simulink model "SVC_Simulation_V2"  (R2024a)
settings: Solver=FixedStepAuto  StartTime=0.0  StopTime=0.6  FixedStep=Ts  MaxStep=1e-5  RelTol=1e-4  AbsTol=1e-4
PreLoadFcn:
  | Ts=50e-6;
model workspace (MAT data in the model file):
  Ki : Simulink.Parameter (value not decoded)
  Kp = 0
symbols that are objects in the model workspace (value not decoded): Ki
undefined symbols (not defined in the file or in its folder): D1, Delta, DiscIntNeverNeededParam, find_system
libraries: spsSampleandHoldLib x24, spsThyristorLib x24, spsEdgeDetectorLib x12, spsSeriesRLCBranchLib x12, spsParallelRLCBranchLib x9, spsBistableLib x3, spsMeanVariableFrequencyLib x3, spsSecondOrderFilterLib x3, spsMultimeterLib x3, spsCurrentMeasurementLib x2, spsThreePhaseVIMeasurementLib x2, spsThreePhaseSeriesRLCLoadLib x1
(part 2 of 3)

== system SVC_Simulation_V2/SVC Controller/Firing Unit/Firing Unit BC ==
  note: PLL
      | sync on
      | pos. peak
      | of input
  note: Generate firing
      | pulses for TSC3
  note: Generate firing
      | pulse for TCR +
  note: Generate firing
      | pulse for TCR -
  note: Generate firing
      | pulses for TSC2
  note: Generate firing
      | pulses for TSC1
  note: Generate square-wave lagging Input
      | voltage by 90 degrees and pulses (width of
      | one sample) for positive (Sync +)
      | and negative (Sync -) transition
  note: Compute number
      | of samples per cycle
  note: Input
      | voltage
  V : Inport  PortDimensions=1
  Alpha : Inport  Port=2  PortDimensions=1
  TSC1_On : Inport  Port=3  PortDimensions=1
  TSC2_On : Inport  Port=4  PortDimensions=1
  TSC3_On : Inport  Port=5  PortDimensions=1
  BL2 : Subsystem
  BL3 : Subsystem
  Correction for delay : Gain  Gain=Nstep*Ts*2*pi  SaturateOnIntegerOverflow=on  OutDataTypeStr=Inherit: Same as input  ParamDataTypeStr=Inherit: Same as input
  Logical Operator2 : Logic  Operator=NOT  Inputs=3
  "PLL sync on positive peak " : Subsystem  mask(Discrete 1-phase PLL){Par_Init=[PhaseInit FreqInit], ParK=[120 2800], Ts=Ts}
      mask prompts: Par_Init "Initial input:[ Phase(degrees)   Frequency(Hz) ]"; ParK "Regulator gains [ Kp  Ki ]"; Ts "Sample time:"
      mask help:
      | This Phase Locked Loop (PLL) system can be used  to synchronize on a variable frequency sinusoidal signal.
      |
      | Input 1: Normalized input signal V(pu)
      mask init:
      | Kp=ParK(1);
      | Ki=ParK(2);
      | Phase_Init=Par_Init(1);
      | Finit=Par_Init(2);
  Sum : Sum  InputSameDT=on  SaturateOnIntegerOverflow=on  OutDataTypeStr=Inherit: Same as first input
  TCR Pulse Generatorr : Subsystem  mask{Ts=Ts}
      mask prompts: Ts "Sample time:"
  TCR Pulse Generatorr1 : Subsystem  mask{Ts=Ts}
      mask prompts: Ts "Sample time:"
  TCS Pulse Generator : Subsystem
  TCS Pulse Generator1 : Subsystem
  TCS Pulse Generator2 : Subsystem
  Trigonometric Function6 : Trigonometry
  TCR + : Outport  VectorParamsAs1DForOutWhenUnconnected=off
  TCR - : Outport  Port=2  VectorParamsAs1DForOutWhenUnconnected=off
  TSC1 + : Outport  Port=3  VectorParamsAs1DForOutWhenUnconnected=off
  TSC1 - : Outport  Port=4  VectorParamsAs1DForOutWhenUnconnected=off
  TSC2 + : Outport  Port=5  VectorParamsAs1DForOutWhenUnconnected=off
  TSC2 - : Outport  Port=6  VectorParamsAs1DForOutWhenUnconnected=off
  TSC3 + : Outport  Port=7  VectorParamsAs1DForOutWhenUnconnected=off
  TSC3 - : Outport  Port=8  VectorParamsAs1DForOutWhenUnconnected=off
  wires:
  Logical Operator2/1 -> TCR Pulse Generatorr1/4(SqWave)
  TCR Pulse Generatorr/1(TCR +/-) -> TCR +/1
  BL3/1(SqWave) -> TCS Pulse Generator/1(SqWave), TCS Pulse Generator2/1(SqWave), TCS Pulse Generator1/1(SqWave), TCR Pulse Generatorr/4(SqWave), Logical Operator2/1
  TCS Pulse Generator2/2(TSC -) -> TSC3 -/1
  TCS Pulse Generator2/1(TSC +) -> TSC3 +/1
  TSC3_On/1 -> TCS Pulse Generator2/4(TSC_On)
  TCR Pulse Generatorr1/1(TCR +/-) -> TCR -/1
  TCS Pulse Generator/2(TSC -) -> TSC1 -/1
  TCS Pulse Generator/1(TSC +) -> TSC1 +/1
  BL3/2(Sync +) -> TCS Pulse Generator2/2(Sync +), TCS Pulse Generator1/2(Sync +), TCS Pulse Generator/2(Sync +), TCR Pulse Generatorr/3(Sync +/-)
  BL3/3(Sync -) -> TCS Pulse Generator/3(Sync -), TCS Pulse Generator2/3(Sync -), TCS Pulse Generator1/3(Sync -), TCR Pulse Generatorr1/3(Sync +/-)
  Alpha/1 -> TCR Pulse Generatorr/2(Alpha), TCR Pulse Generatorr1/2(Alpha)
  TSC1_On/1 -> TCS Pulse Generator/4(TSC_On)
  TCS Pulse Generator1/2(TSC -) -> TSC2 -/1
  TCS Pulse Generator1/1(TSC +) -> TSC2 +/1
  TSC2_On/1 -> TCS Pulse Generator1/4(TSC_On)
  BL2/1(Ns/c) -> TCR Pulse Generatorr/1(Ns/c), TCR Pulse Generatorr1/1(Ns/c)
  "PLL sync on positive peak "/2(wt) -> Sum/2
  Sum/1 -> Trigonometric Function6/1
  Trigonometric Function6/1 -> BL3/2(sin(wt))
  Correction for delay/1 -> Sum/1
  "PLL sync on positive peak "/1(Freq) -> BL2/1(Freq), BL3/1(Freq), Correction for delay/1
  V/1 -> "PLL sync on positive peak "/1(V(pu))

== system SVC_Simulation_V2/SVC Controller/Firing Unit/Firing Unit CA ==
  note: PLL
      | sync on
      | pos. peak
      | of input
  note: Generate firing
      | pulses for TSC3
  note: Generate firing
      | pulse for TCR +
  note: Generate firing
      | pulse for TCR -
  note: Generate firing
      | pulses for TSC2
  note: Generate firing
      | pulses for TSC1
  note: Generate square-wave lagging Input
      | voltage by 90 degrees and pulses (width of
      | one sample) for positive (Sync +)
      | and negative (Sync -) transition
  note: Compute number
      | of samples per cycle
  note: Input
      | voltage
  V : Inport  PortDimensions=1
  Alpha : Inport  Port=2  PortDimensions=1
  TSC1_On : Inport  Port=3  PortDimensions=1
  TSC2_On : Inport  Port=4  PortDimensions=1
  TSC3_On : Inport  Port=5  PortDimensions=1
  BL2 : Subsystem
  BL3 : Subsystem
  Correction for delay : Gain  Gain=Nstep*Ts*2*pi  SaturateOnIntegerOverflow=on  OutDataTypeStr=Inherit: Same as input  ParamDataTypeStr=Inherit: Same as input
  Logical Operator2 : Logic  Operator=NOT  Inputs=3
  "PLL sync on positive peak " : Subsystem  mask(Discrete 1-phase PLL){Par_Init=[PhaseInit FreqInit], ParK=[120 2800], Ts=Ts}
      mask prompts: Par_Init "Initial input:[ Phase(degrees)   Frequency(Hz) ]"; ParK "Regulator gains [ Kp  Ki ]"; Ts "Sample time:"
      mask help:
      | This Phase Locked Loop (PLL) system can be used  to synchronize on a variable frequency sinusoidal signal.
      |
      | Input 1: Normalized input signal V(pu)
      mask init:
      | Kp=ParK(1);
      | Ki=ParK(2);
      | Phase_Init=Par_Init(1);
      | Finit=Par_Init(2);
  Sum : Sum  InputSameDT=on  SaturateOnIntegerOverflow=on  OutDataTypeStr=Inherit: Same as first input
  TCR Pulse Generatorr : Subsystem  mask{Ts=Ts}
      mask prompts: Ts "Sample time:"
  TCR Pulse Generatorr1 : Subsystem  mask{Ts=Ts}
      mask prompts: Ts "Sample time:"
  TCS Pulse Generator : Subsystem
  TCS Pulse Generator1 : Subsystem
  TCS Pulse Generator2 : Subsystem
  Trigonometric Function6 : Trigonometry
  TCR + : Outport  VectorParamsAs1DForOutWhenUnconnected=off
  TCR - : Outport  Port=2  VectorParamsAs1DForOutWhenUnconnected=off
  TSC1 + : Outport  Port=3  VectorParamsAs1DForOutWhenUnconnected=off
  TSC1 - : Outport  Port=4  VectorParamsAs1DForOutWhenUnconnected=off
  TSC2 + : Outport  Port=5  VectorParamsAs1DForOutWhenUnconnected=off
  TSC2 - : Outport  Port=6  VectorParamsAs1DForOutWhenUnconnected=off
  TSC3 + : Outport  Port=7  VectorParamsAs1DForOutWhenUnconnected=off
  TSC3 - : Outport  Port=8  VectorParamsAs1DForOutWhenUnconnected=off
  wires:
  Logical Operator2/1 -> TCR Pulse Generatorr1/4(SqWave)
  TCR Pulse Generatorr/1(TCR +/-) -> TCR +/1
  BL3/1(SqWave) -> TCS Pulse Generator/1(SqWave), TCS Pulse Generator2/1(SqWave), TCS Pulse Generator1/1(SqWave), TCR Pulse Generatorr/4(SqWave), Logical Operator2/1
  TCS Pulse Generator2/2(TSC -) -> TSC3 -/1
  TCS Pulse Generator2/1(TSC +) -> TSC3 +/1
  TSC3_On/1 -> TCS Pulse Generator2/4(TSC_On)
  TCR Pulse Generatorr1/1(TCR +/-) -> TCR -/1
  TCS Pulse Generator/2(TSC -) -> TSC1 -/1
  TCS Pulse Generator/1(TSC +) -> TSC1 +/1
  BL3/2(Sync +) -> TCS Pulse Generator2/2(Sync +), TCS Pulse Generator1/2(Sync +), TCS Pulse Generator/2(Sync +), TCR Pulse Generatorr/3(Sync +/-)
  BL3/3(Sync -) -> TCS Pulse Generator/3(Sync -), TCS Pulse Generator2/3(Sync -), TCS Pulse Generator1/3(Sync -), TCR Pulse Generatorr1/3(Sync +/-)
  Alpha/1 -> TCR Pulse Generatorr/2(Alpha), TCR Pulse Generatorr1/2(Alpha)
  TSC1_On/1 -> TCS Pulse Generator/4(TSC_On)
  TCS Pulse Generator1/2(TSC -) -> TSC2 -/1
  TCS Pulse Generator1/1(TSC +) -> TSC2 +/1
  TSC2_On/1 -> TCS Pulse Generator1/4(TSC_On)
  BL2/1(Ns/c) -> TCR Pulse Generatorr/1(Ns/c), TCR Pulse Generatorr1/1(Ns/c)
  "PLL sync on positive peak "/2(wt) -> Sum/2
  Sum/1 -> Trigonometric Function6/1
  Trigonometric Function6/1 -> BL3/2(sin(wt))
  Correction for delay/1 -> Sum/1
  "PLL sync on positive peak "/1(Freq) -> BL2/1(Freq), BL3/1(Freq), Correction for delay/1
  V/1 -> "PLL sync on positive peak "/1(V(pu))

== system SVC_Simulation_V2/SVC Controller/Firing Unit/Firing Unit AB/BL2 ==
  Freq : Inport  PortDimensions=1
  Constant1 : Constant  Value=0
  Constant2 : Constant  Value=1e-5
  Constant3 : Constant
  Gain : Gain  Gain=Ts  SaturateOnIntegerOverflow=on  OutDataTypeStr=Inherit: Same as input  ParamDataTypeStr=Inherit: Same as input
  Product : Product  Inputs=/*  InputSameDT=on  SaturateOnIntegerOverflow=on  OutDataTypeStr=Inherit: Same as first input
  Relational Operator1 : RelationalOperator  Operator=~=
  Switch : Switch  Threshold=0.5
  Ns/c : Outport  VectorParamsAs1DForOutWhenUnconnected=off
  wires:
  Product/1 -> Ns/c/1
  Freq/1 -> Gain/1
  Constant1/1 -> Relational Operator1/2
  Gain/1 -> Relational Operator1/1, Switch/1
  Constant2/1 -> Switch/3
  Relational Operator1/1 -> Switch/2
  Switch/1 -> Product/1
  Constant3/1 -> Product/2

== system SVC_Simulation_V2/SVC Controller/Firing Unit/Firing Unit AB/BL3 ==
  Freq : Inport  PortDimensions=1
  sin(wt) : Inport  Port=2  PortDimensions=1
  Bistable : spsBistableLib/Bistable  Qpriority=Set  ic=0  Ts=Ts
  Data Type Conversion : DataTypeConversion  SaturateOnIntegerOverflow=off  RndMeth=Floor
  Edge Detector : spsEdgeDetectorLib/Edge Detector  model=Rising  ic=0  Ts=Ts
  Edge Detector1 : spsEdgeDetectorLib/Edge Detector  model=Falling  ic=0  Ts=Ts
  Edge Detector2 : spsEdgeDetectorLib/Edge Detector  model=Rising  ic=0  Ts=Ts
  Edge Detector3 : spsEdgeDetectorLib/Edge Detector  model=Rising  ic=0  Ts=Ts
  Product2 : Product  InputSameDT=on  SaturateOnIntegerOverflow=on  OutDataTypeStr=Inherit: Same as first input
  Relational Operator : RelationalOperator  Operator=>
  Relational Operator2 : RelationalOperator  Operator=<
  Sum5 : Sum  Inputs=+-  InputSameDT=on  SaturateOnIntegerOverflow=on  OutDataTypeStr=Inherit: Same as first input
  Sum6 : Sum  InputSameDT=on  SaturateOnIntegerOverflow=on  OutDataTypeStr=Inherit: Same as first input
  Terminator : Terminator
  Trigonometric Function7 : Trigonometry
  alpha2 : Constant  Value=0
  alpha9 : Constant  Value=pi*Ts
  SqWave : Outport  VectorParamsAs1DForOutWhenUnconnected=off
  Sync + : Outport  Port=2  VectorParamsAs1DForOutWhenUnconnected=off
  Sync - : Outport  Port=3  VectorParamsAs1DForOutWhenUnconnected=off
  wires:
  Data Type Conversion/1 -> Edge Detector/1, Edge Detector1/1, SqWave/1
  Bistable/2 -> Terminator/1
  Edge Detector3/1 -> Bistable/2
  Edge Detector2/1 -> Bistable/1
  Edge Detector1/1 -> Sync -/1
  Edge Detector/1 -> Sync +/1
  Bistable/1 -> Data Type Conversion/1
  alpha9/1 -> Product2/1
  Product2/1 -> Trigonometric Function7/1
  Relational Operator2/1 -> Edge Detector3/1
  Relational Operator/1 -> Edge Detector2/1
  Sum6/1 -> Relational Operator2/2
  Sum5/1 -> Relational Operator/2
  alpha2/1 -> Sum6/1, Sum5/1
  Trigonometric Function7/1 -> Sum6/2, Sum5/2
  Freq/1 -> Product2/2
  sin(wt)/1 -> Relational Operator/1, Relational Operator2/1

== system SVC_Simulation_V2/SVC Controller/Firing Unit/Firing Unit AB/PLL sync on positive peak  ==
  note: Note: -sin( a ) * sin( b ) = 1/2 * cos( a+b ) - 1/2 * cos(a-b)
  note: Discrete 1-phase PLL
  note: Note: PLL synchronized on positive peak of input
  note: Pierre Giroux, Gilbert Sybille
      | Power System Laboratory, IREQ
      | Hydro-Quebec
  V(pu) : Inport
  Constant4 : Constant  Value=2*pi
  Discrete PI Controller : Subsystem  DialogController=POWERSYS.PowerSysDialog  mask(Discrete PI Controller){Kp=Kp, Ki=Ki, Par_Limits=[1.25  0.75]*2*pi*Finit, Init=2*pi*Finit, Ts=Ts}
      mask prompts: Kp "Proportional gain (Kp):"; Ki "Integral gain (Ki):"; Par_Limits "Output limits: [ Upper   Lower ]"; Init "Output initial value:"; Ts "Sample time:"
      mask help: This block implements a discrete PI controller.
      mask init:
      | UpperLimit=Par_Limits(1);
      | LowerLimit=Par_Limits(2);
      | power_initmask();
      mask Help: This block is part of a subset of blocks in the Extras library that does not have documentation associated with it, other than the block mask description.
      mask Display: disp('PI');
  Discrete-Time Integrator : DiscreteIntegrator  InitialCondition=(Phase_Init-90)*pi/180  SampleTime=Ts  ICPrevOutput=DiscIntNeverNeededParam  ICPrevScaledInput=DiscIntNeverNeededParam
  Gain10 : Gain  Gain=1/2/pi  SaturateOnIntegerOverflow=on  OutDataTypeStr=Inherit: Same as input  ParamDataTypeStr=Inherit: Same as input
  Gain12 : Gain  Gain=-1  SaturateOnIntegerOverflow=on  OutDataTypeStr=Inherit: Same as input  ParamDataTypeStr=Inherit: Same as input
  Math Function : Math  Operator=mod  SignedPower=on
  Mean (Variable Frequency)1 : spsMeanVariableFrequencyLib/Mean (Variable Frequency)  Finit=Finit  Fmin=45  Vinit=0  Ts=Ts
  Product1 : Product  InputSameDT=on  SaturateOnIntegerOverflow=on  OutDataTypeStr=Inherit: Same as first input
  Rate Limiter : RateLimiter  RisingSlewLimit=10  FallingSlewLimit=-10  SampleTimeMode=inherited  InitialCondition=Finit
  Second-Order Filter : spsSecondOrderFilterLib/Second-Order Filter  FilterType=Lowpass  Fo=25  Zeta=0.707  Ts=Ts  Initialize=on  Vac_Init="[0 0  Finit]"  Vdc_Init=Finit  PlotResponse=off  FreqRange=[1 500 1]
  Trigonometric Function6 : Trigonometry
  Unit Delay1 : UnitDelay  InitialCondition=Finit  SampleTime=Ts  HasFrameUpgradeWarning=on
      settings: AttributesFormatString=IC = %<InitialCondition>
  Freq : Outport  VectorParamsAs1DForOutWhenUnconnected=off
  wt : Outport  Port=2  VectorParamsAs1DForOutWhenUnconnected=off
  wires:
  Gain12/1 -> Product1/1
  V(pu)/1 -> Gain12/1
  Constant4/1 -> Math Function/2
  Discrete-Time Integrator/1 -> Math Function/1
  Product1/1 -> Mean (Variable Frequency)1/2
  Discrete PI Controller/1(Out) -> Discrete-Time Integrator/1, Gain10/1  "W"
  Gain10/1 -> Rate Limiter/1
  Rate Limiter/1 -> Second-Order Filter/1
  Second-Order Filter/1 -> Unit Delay1/1
  Trigonometric Function6/1 -> Product1/2
  Math Function/1 -> Trigonometric Function6/1, wt/1
  Unit Delay1/1 -> Mean (Variable Frequency)1/1, Freq/1
  Mean (Variable Frequency)1/1 -> Discrete PI Controller/1(Error)

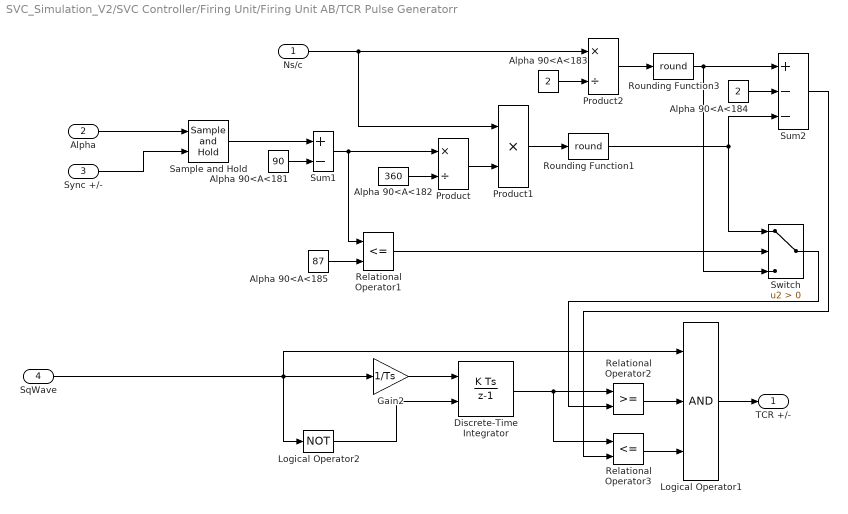
== system SVC_Simulation_V2/SVC Controller/Firing Unit/Firing Unit AB/TCR Pulse Generatorr ==
  Ns/c : Inport
  Alpha : Inport  Port=2  PortDimensions=1
  Sync +/- : Inport  Port=3  PortDimensions=1
  SqWave : Inport  Port=4  PortDimensions=1
  Alpha 90<A<181 : Constant  Value=90
  Alpha 90<A<182 : Constant  Value=360
  Alpha 90<A<183 : Constant  Value=2
  Alpha 90<A<184 : Constant  Value=2
  Alpha 90<A<185 : Constant  Value=87
  Discrete-Time Integrator : DiscreteIntegrator  ExternalReset=rising  SampleTime=Ts  LimitOutput=on  UpperSaturationLimit=100000  LowerSaturationLimit=0  ICPrevOutput=DiscIntNeverNeededParam  ICPrevScaledInput=DiscIntNeverNeededParam
  Gain2 : Gain  Gain=1/Ts  SaturateOnIntegerOverflow=on  OutDataTypeStr=Inherit: Same as input  ParamDataTypeStr=Inherit: Same as input
  Logical Operator1 : Logic  Inputs=3
  Logical Operator2 : Logic  Operator=NOT  Inputs=3
  Product : Product  Inputs=*/  InputSameDT=on  SaturateOnIntegerOverflow=on  OutDataTypeStr=Inherit: Same as first input
  Product1 : Product  Inputs=**  InputSameDT=on  SaturateOnIntegerOverflow=on  OutDataTypeStr=Inherit: Same as first input
  Product2 : Product  Inputs=*/  InputSameDT=on  SaturateOnIntegerOverflow=on  OutDataTypeStr=Inherit: Same as first input
  Relational Operator1 : RelationalOperator  Operator=<=
  Relational Operator2 : RelationalOperator
  Relational Operator3 : RelationalOperator  Operator=<=
  Rounding Function1 : Rounding  Operator=round
  Rounding Function3 : Rounding  Operator=round
  Sample and Hold : spsSampleandHoldLib/Sample and Hold  ic=180  Ts=Ts
      settings: AttributesFormatString=IC = %<ic>
  Sum1 : Sum  Inputs=+-  InputSameDT=on  SaturateOnIntegerOverflow=on  OutDataTypeStr=Inherit: Same as first input
  Sum2 : Sum  Inputs=+--  InputSameDT=on  SaturateOnIntegerOverflow=on  OutDataTypeStr=Inherit: Same as first input
  Switch : Switch  Criteria=u2 > Threshold
  TCR +/- : Outport  VectorParamsAs1DForOutWhenUnconnected=off
  wires:
  Alpha 90<A<181/1 -> Sum1/2
  Ns/c/1 -> Product1/1, Product2/1
  Product1/1 -> Rounding Function1/1
  Alpha 90<A<182/1 -> Product/2
  Product/1 -> Product1/2
  Product2/1 -> Rounding Function3/1
  Alpha 90<A<183/1 -> Product2/2
  Sum1/1 -> Product/1, Relational Operator1/1
  Alpha 90<A<185/1 -> Relational Operator1/2
  Alpha/1 -> Sample and Hold/1
  Rounding Function1/1 -> Sum2/3, Switch/1
  Rounding Function3/1 -> Sum2/1, Switch/3
  Alpha 90<A<184/1 -> Sum2/2
  Relational Operator1/1 -> Switch/2
  Relational Operator3/1 -> Logical Operator1/3
  Discrete-Time Integrator/1 -> Relational Operator2/1, Relational Operator3/1
  Relational Operator2/1 -> Logical Operator1/2
  Logical Operator1/1 -> TCR +/-/1
  Gain2/1 -> Discrete-Time Integrator/1
  Switch/1 -> Relational Operator2/2
  Sum2/1 -> Relational Operator3/2
  Logical Operator2/1 -> Discrete-Time Integrator/2
  SqWave/1 -> Gain2/1, Logical Operator2/1, Logical Operator1/1
  Sync +/-/1 -> Sample and Hold/2
  Sample and Hold/1 -> Sum1/1

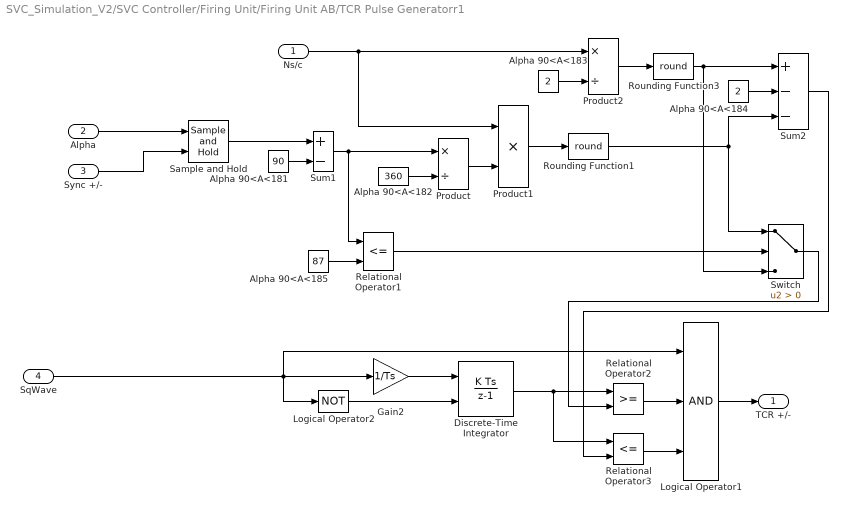
== system SVC_Simulation_V2/SVC Controller/Firing Unit/Firing Unit AB/TCR Pulse Generatorr1 ==
  Ns/c : Inport
  Alpha : Inport  Port=2  PortDimensions=1
  Sync +/- : Inport  Port=3  PortDimensions=1
  SqWave : Inport  Port=4  PortDimensions=1
  Alpha 90<A<181 : Constant  Value=90
  Alpha 90<A<182 : Constant  Value=360
  Alpha 90<A<183 : Constant  Value=2
  Alpha 90<A<184 : Constant  Value=2
  Alpha 90<A<185 : Constant  Value=87
  Discrete-Time Integrator : DiscreteIntegrator  ExternalReset=rising  SampleTime=Ts  LimitOutput=on  UpperSaturationLimit=100000  LowerSaturationLimit=0  ICPrevOutput=DiscIntNeverNeededParam  ICPrevScaledInput=DiscIntNeverNeededParam
  Gain2 : Gain  Gain=1/Ts  SaturateOnIntegerOverflow=on  OutDataTypeStr=Inherit: Same as input  ParamDataTypeStr=Inherit: Same as input
  Logical Operator1 : Logic  Inputs=3
  Logical Operator2 : Logic  Operator=NOT  Inputs=3
  Product : Product  Inputs=*/  InputSameDT=on  SaturateOnIntegerOverflow=on  OutDataTypeStr=Inherit: Same as first input
  Product1 : Product  Inputs=**  InputSameDT=on  SaturateOnIntegerOverflow=on  OutDataTypeStr=Inherit: Same as first input
  Product2 : Product  Inputs=*/  InputSameDT=on  SaturateOnIntegerOverflow=on  OutDataTypeStr=Inherit: Same as first input
  Relational Operator1 : RelationalOperator  Operator=<=
  Relational Operator2 : RelationalOperator
  Relational Operator3 : RelationalOperator  Operator=<=
  Rounding Function1 : Rounding  Operator=round
  Rounding Function3 : Rounding  Operator=round
  Sample and Hold : spsSampleandHoldLib/Sample and Hold  ic=180  Ts=Ts
      settings: AttributesFormatString=IC = %<ic>
  Sum1 : Sum  Inputs=+-  InputSameDT=on  SaturateOnIntegerOverflow=on  OutDataTypeStr=Inherit: Same as first input
  Sum2 : Sum  Inputs=+--  InputSameDT=on  SaturateOnIntegerOverflow=on  OutDataTypeStr=Inherit: Same as first input
  Switch : Switch  Criteria=u2 > Threshold
  TCR +/- : Outport  VectorParamsAs1DForOutWhenUnconnected=off
  wires:
  Alpha 90<A<181/1 -> Sum1/2
  Ns/c/1 -> Product1/1, Product2/1
  Product1/1 -> Rounding Function1/1
  Alpha 90<A<182/1 -> Product/2
  Product/1 -> Product1/2
  Product2/1 -> Rounding Function3/1
  Alpha 90<A<183/1 -> Product2/2
  Sum1/1 -> Product/1, Relational Operator1/1
  Alpha 90<A<185/1 -> Relational Operator1/2
  Alpha/1 -> Sample and Hold/1
  Rounding Function1/1 -> Sum2/3, Switch/1
  Rounding Function3/1 -> Sum2/1, Switch/3
  Alpha 90<A<184/1 -> Sum2/2
  Relational Operator1/1 -> Switch/2
  Relational Operator3/1 -> Logical Operator1/3
  Discrete-Time Integrator/1 -> Relational Operator2/1, Relational Operator3/1
  Relational Operator2/1 -> Logical Operator1/2
  Logical Operator1/1 -> TCR +/-/1
  Gain2/1 -> Discrete-Time Integrator/1
  Switch/1 -> Relational Operator2/2
  Sum2/1 -> Relational Operator3/2
  Logical Operator2/1 -> Discrete-Time Integrator/2
  SqWave/1 -> Gain2/1, Logical Operator2/1, Logical Operator1/1
  Sync +/-/1 -> Sample and Hold/2
  Sample and Hold/1 -> Sum1/1

== system SVC_Simulation_V2/SVC Controller/Firing Unit/Firing Unit AB/TCS Pulse Generator ==
  note: Note: Sync+ , Sync - and SqWave signals are inverted for TSC firing (i.e. positive thyristor is fired on negative peak voltage)
  SqWave : Inport  PortDimensions=1
  Sync + : Inport  Port=2  PortDimensions=1
  Sync - : Inport  Port=3  PortDimensions=1
  TSC_On : Inport  Port=4  PortDimensions=1
  Alpha1 : Constant  Value=FiringMode-1
  Delay : Delay  DelayLength=fix(1/FreqInit/Ts)
  Logical Operator1 : Logic  Operator=NOT
  Logical Operator10 : Logic  Operator=OR
  Logical Operator11 : Logic  Inputs=3
  Logical Operator12 : Logic
  Logical Operator13 : Logic
  Logical Operator14 : Logic  Operator=OR
  Logical Operator15 : Logic  Inputs=3
  Sample and Hold : spsSampleandHoldLib/Sample and Hold  ic=0  Ts=Ts
      settings: AttributesFormatString=IC = %<ic>
  Sample and Hold1 : spsSampleandHoldLib/Sample and Hold  ic=0  Ts=Ts
      settings: AttributesFormatString=IC = %<ic>
  TSC + : Outport  VectorParamsAs1DForOutWhenUnconnected=off
  TSC - : Outport  Port=2  VectorParamsAs1DForOutWhenUnconnected=off
  wires:
  Delay/1 -> Logical Operator14/2, Logical Operator10/2
  Logical Operator15/1 -> TSC -/1
  Logical Operator11/1 -> TSC +/1
  Logical Operator14/1 -> Logical Operator15/2
  Logical Operator10/1 -> Logical Operator11/2
  Logical Operator1/1 -> Logical Operator10/1
  SqWave/1 -> Logical Operator14/1, Logical Operator1/1
  Logical Operator12/1 -> Delay/1
  Alpha1/1 -> Logical Operator12/2
  Logical Operator13/1 -> Logical Operator12/1
  TSC_On/1 -> Sample and Hold1/1, Sample and Hold/1, Logical Operator15/3, Logical Operator11/3
  Sync -/1 -> Sample and Hold/2
  Sync +/1 -> Sample and Hold1/2
  Sample and Hold/1 -> Logical Operator13/1, Logical Operator11/1
  Sample and Hold1/1 -> Logical Operator13/2, Logical Operator15/1

== system SVC_Simulation_V2/SVC Controller/Firing Unit/Firing Unit AB/TCS Pulse Generator1 ==
  note: Note: Sync+ , Sync - and SqWave signals are inverted for TSC firing (i.e. positive thyristor is fired on negative peak voltage)
  SqWave : Inport  PortDimensions=1
  Sync + : Inport  Port=2  PortDimensions=1
  Sync - : Inport  Port=3  PortDimensions=1
  TSC_On : Inport  Port=4  PortDimensions=1
  Alpha1 : Constant  Value=FiringMode-1
  Delay : Delay  DelayLength=fix(1/FreqInit/Ts)
  Logical Operator1 : Logic  Operator=NOT
  Logical Operator10 : Logic  Operator=OR
  Logical Operator11 : Logic  Inputs=3
  Logical Operator12 : Logic
  Logical Operator13 : Logic
  Logical Operator14 : Logic  Operator=OR
  Logical Operator15 : Logic  Inputs=3
  Sample and Hold : spsSampleandHoldLib/Sample and Hold  ic=0  Ts=Ts
      settings: AttributesFormatString=IC = %<ic>
  Sample and Hold1 : spsSampleandHoldLib/Sample and Hold  ic=0  Ts=Ts
      settings: AttributesFormatString=IC = %<ic>
  TSC + : Outport  VectorParamsAs1DForOutWhenUnconnected=off
  TSC - : Outport  Port=2  VectorParamsAs1DForOutWhenUnconnected=off
  wires:
  Delay/1 -> Logical Operator14/2, Logical Operator10/2
  Logical Operator15/1 -> TSC -/1
  Logical Operator11/1 -> TSC +/1
  Logical Operator14/1 -> Logical Operator15/2
  Logical Operator10/1 -> Logical Operator11/2
  Logical Operator1/1 -> Logical Operator10/1
  SqWave/1 -> Logical Operator14/1, Logical Operator1/1
  Logical Operator12/1 -> Delay/1
  Alpha1/1 -> Logical Operator12/2
  Logical Operator13/1 -> Logical Operator12/1
  TSC_On/1 -> Sample and Hold1/1, Sample and Hold/1, Logical Operator15/3, Logical Operator11/3
  Sync -/1 -> Sample and Hold/2
  Sync +/1 -> Sample and Hold1/2
  Sample and Hold/1 -> Logical Operator13/1, Logical Operator11/1
  Sample and Hold1/1 -> Logical Operator13/2, Logical Operator15/1

== system SVC_Simulation_V2/SVC Controller/Firing Unit/Firing Unit AB/TCS Pulse Generator2 ==
  note: Note: Sync+ , Sync - and SqWave signals are inverted for TSC firing (i.e. positive thyristor is fired on negative peak voltage)
  SqWave : Inport  PortDimensions=1
  Sync + : Inport  Port=2  PortDimensions=1
  Sync - : Inport  Port=3  PortDimensions=1
  TSC_On : Inport  Port=4  PortDimensions=1
  Alpha1 : Constant  Value=FiringMode-1
  Delay : Delay  DelayLength=fix(1/FreqInit/Ts)
  Logical Operator1 : Logic  Operator=NOT
  Logical Operator10 : Logic  Operator=OR
  Logical Operator11 : Logic  Inputs=3
  Logical Operator12 : Logic
  Logical Operator13 : Logic
  Logical Operator14 : Logic  Operator=OR
  Logical Operator15 : Logic  Inputs=3
  Sample and Hold : spsSampleandHoldLib/Sample and Hold  ic=0  Ts=Ts
      settings: AttributesFormatString=IC = %<ic>
  Sample and Hold1 : spsSampleandHoldLib/Sample and Hold  ic=0  Ts=Ts
      settings: AttributesFormatString=IC = %<ic>
  TSC + : Outport  VectorParamsAs1DForOutWhenUnconnected=off
  TSC - : Outport  Port=2  VectorParamsAs1DForOutWhenUnconnected=off
  wires:
  Delay/1 -> Logical Operator14/2, Logical Operator10/2
  Logical Operator15/1 -> TSC -/1
  Logical Operator11/1 -> TSC +/1
  Logical Operator14/1 -> Logical Operator15/2
  Logical Operator10/1 -> Logical Operator11/2
  Logical Operator1/1 -> Logical Operator10/1
  SqWave/1 -> Logical Operator14/1, Logical Operator1/1
  Logical Operator12/1 -> Delay/1
  Alpha1/1 -> Logical Operator12/2
  Logical Operator13/1 -> Logical Operator12/1
  TSC_On/1 -> Sample and Hold1/1, Sample and Hold/1, Logical Operator15/3, Logical Operator11/3
  Sync -/1 -> Sample and Hold/2
  Sync +/1 -> Sample and Hold1/2
  Sample and Hold/1 -> Logical Operator13/1, Logical Operator11/1
  Sample and Hold1/1 -> Logical Operator13/2, Logical Operator15/1

== system SVC_Simulation_V2/SVC Controller/Firing Unit/Firing Unit BC/BL2 ==
  Freq : Inport  PortDimensions=1
  Constant1 : Constant  Value=0
  Constant2 : Constant  Value=1e-5
  Constant3 : Constant
  Gain : Gain  Gain=Ts  SaturateOnIntegerOverflow=on  OutDataTypeStr=Inherit: Same as input  ParamDataTypeStr=Inherit: Same as input
  Product : Product  Inputs=/*  InputSameDT=on  SaturateOnIntegerOverflow=on  OutDataTypeStr=Inherit: Same as first input
  Relational Operator1 : RelationalOperator  Operator=~=
  Switch : Switch  Threshold=0.5
  Ns/c : Outport  VectorParamsAs1DForOutWhenUnconnected=off
  wires:
  Product/1 -> Ns/c/1
  Freq/1 -> Gain/1
  Constant1/1 -> Relational Operator1/2
  Gain/1 -> Relational Operator1/1, Switch/1
  Constant2/1 -> Switch/3
  Relational Operator1/1 -> Switch/2
  Switch/1 -> Product/1
  Constant3/1 -> Product/2

== system SVC_Simulation_V2/SVC Controller/Firing Unit/Firing Unit BC/BL3 ==
  Freq : Inport  PortDimensions=1
  sin(wt) : Inport  Port=2  PortDimensions=1
  Bistable : spsBistableLib/Bistable  Qpriority=Set  ic=0  Ts=Ts
  Data Type Conversion : DataTypeConversion  SaturateOnIntegerOverflow=off  RndMeth=Floor
  Edge Detector : spsEdgeDetectorLib/Edge Detector  model=Rising  ic=0  Ts=Ts
  Edge Detector1 : spsEdgeDetectorLib/Edge Detector  model=Falling  ic=0  Ts=Ts
  Edge Detector2 : spsEdgeDetectorLib/Edge Detector  model=Rising  ic=0  Ts=Ts
  Edge Detector3 : spsEdgeDetectorLib/Edge Detector  model=Rising  ic=0  Ts=Ts
  Product2 : Product  InputSameDT=on  SaturateOnIntegerOverflow=on  OutDataTypeStr=Inherit: Same as first input
  Relational Operator : RelationalOperator  Operator=>
  Relational Operator2 : RelationalOperator  Operator=<
  Sum5 : Sum  Inputs=+-  InputSameDT=on  SaturateOnIntegerOverflow=on  OutDataTypeStr=Inherit: Same as first input
  Sum6 : Sum  InputSameDT=on  SaturateOnIntegerOverflow=on  OutDataTypeStr=Inherit: Same as first input
  Terminator : Terminator
  Trigonometric Function7 : Trigonometry
  alpha2 : Constant  Value=0
  alpha9 : Constant  Value=pi*Ts
  SqWave : Outport  VectorParamsAs1DForOutWhenUnconnected=off
  Sync + : Outport  Port=2  VectorParamsAs1DForOutWhenUnconnected=off
  Sync - : Outport  Port=3  VectorParamsAs1DForOutWhenUnconnected=off
  wires:
  Data Type Conversion/1 -> Edge Detector/1, Edge Detector1/1, SqWave/1
  Bistable/2 -> Terminator/1
  Edge Detector3/1 -> Bistable/2
  Edge Detector2/1 -> Bistable/1
  Edge Detector1/1 -> Sync -/1
  Edge Detector/1 -> Sync +/1
  Bistable/1 -> Data Type Conversion/1
  alpha9/1 -> Product2/1
  Product2/1 -> Trigonometric Function7/1
  Relational Operator2/1 -> Edge Detector3/1
  Relational Operator/1 -> Edge Detector2/1
  Sum6/1 -> Relational Operator2/2
  Sum5/1 -> Relational Operator/2
  alpha2/1 -> Sum6/1, Sum5/1
  Trigonometric Function7/1 -> Sum6/2, Sum5/2
  Freq/1 -> Product2/2
  sin(wt)/1 -> Relational Operator/1, Relational Operator2/1

== system SVC_Simulation_V2/SVC Controller/Firing Unit/Firing Unit BC/PLL sync on positive peak  ==
  note: Note: -sin( a ) * sin( b ) = 1/2 * cos( a+b ) - 1/2 * cos(a-b)
  note: Discrete 1-phase PLL
  note: Note: PLL synchronized on positive peak of input
  note: Pierre Giroux, Gilbert Sybille
      | Power System Laboratory, IREQ
      | Hydro-Quebec
  V(pu) : Inport
  Constant4 : Constant  Value=2*pi
  Discrete PI Controller : Subsystem  DialogController=POWERSYS.PowerSysDialog  mask(Discrete PI Controller){Kp=Kp, Ki=Ki, Par_Limits=[1.25  0.75]*2*pi*Finit, Init=2*pi*Finit, Ts=Ts}
      mask prompts: Kp "Proportional gain (Kp):"; Ki "Integral gain (Ki):"; Par_Limits "Output limits: [ Upper   Lower ]"; Init "Output initial value:"; Ts "Sample time:"
      mask help: This block implements a discrete PI controller.
      mask init:
      | UpperLimit=Par_Limits(1);
      | LowerLimit=Par_Limits(2);
      | power_initmask();
      mask Help: This block is part of a subset of blocks in the Extras library that does not have documentation associated with it, other than the block mask description.
      mask Display: disp('PI');
  Discrete-Time Integrator : DiscreteIntegrator  InitialCondition=(Phase_Init-90)*pi/180  SampleTime=Ts  ICPrevOutput=DiscIntNeverNeededParam  ICPrevScaledInput=DiscIntNeverNeededParam
  Gain10 : Gain  Gain=1/2/pi  SaturateOnIntegerOverflow=on  OutDataTypeStr=Inherit: Same as input  ParamDataTypeStr=Inherit: Same as input
  Gain12 : Gain  Gain=-1  SaturateOnIntegerOverflow=on  OutDataTypeStr=Inherit: Same as input  ParamDataTypeStr=Inherit: Same as input
  Math Function : Math  Operator=mod  SignedPower=on
  Mean (Variable Frequency)1 : spsMeanVariableFrequencyLib/Mean (Variable Frequency)  Finit=Finit  Fmin=45  Vinit=0  Ts=Ts
  Product1 : Product  InputSameDT=on  SaturateOnIntegerOverflow=on  OutDataTypeStr=Inherit: Same as first input
  Rate Limiter : RateLimiter  RisingSlewLimit=10  FallingSlewLimit=-10  SampleTimeMode=inherited  InitialCondition=Finit
  Second-Order Filter : spsSecondOrderFilterLib/Second-Order Filter  FilterType=Lowpass  Fo=25  Zeta=0.707  Ts=Ts  Initialize=on  Vac_Init="[0 0  Finit]"  Vdc_Init=Finit  PlotResponse=off  FreqRange=[1 500 1]
  Trigonometric Function6 : Trigonometry
  Unit Delay1 : UnitDelay  InitialCondition=Finit  SampleTime=Ts  HasFrameUpgradeWarning=on
      settings: AttributesFormatString=IC = %<InitialCondition>
  Freq : Outport  VectorParamsAs1DForOutWhenUnconnected=off
  wt : Outport  Port=2  VectorParamsAs1DForOutWhenUnconnected=off
  wires:
  Gain12/1 -> Product1/1
  V(pu)/1 -> Gain12/1
  Constant4/1 -> Math Function/2
  Discrete-Time Integrator/1 -> Math Function/1
  Product1/1 -> Mean (Variable Frequency)1/2
  Discrete PI Controller/1(Out) -> Discrete-Time Integrator/1, Gain10/1  "W"
  Gain10/1 -> Rate Limiter/1
  Rate Limiter/1 -> Second-Order Filter/1
  Second-Order Filter/1 -> Unit Delay1/1
  Trigonometric Function6/1 -> Product1/2
  Math Function/1 -> Trigonometric Function6/1, wt/1
  Unit Delay1/1 -> Mean (Variable Frequency)1/1, Freq/1
  Mean (Variable Frequency)1/1 -> Discrete PI Controller/1(Error)

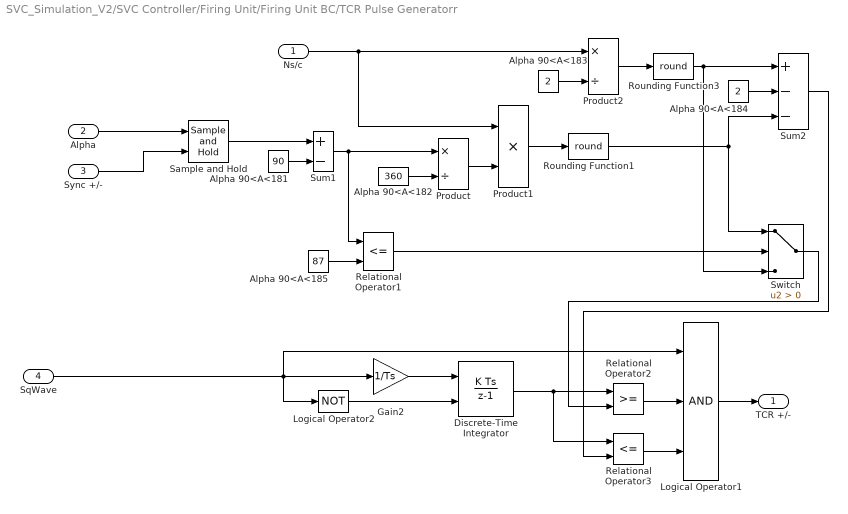
== system SVC_Simulation_V2/SVC Controller/Firing Unit/Firing Unit BC/TCR Pulse Generatorr ==
  Ns/c : Inport
  Alpha : Inport  Port=2  PortDimensions=1
  Sync +/- : Inport  Port=3  PortDimensions=1
  SqWave : Inport  Port=4  PortDimensions=1
  Alpha 90<A<181 : Constant  Value=90
  Alpha 90<A<182 : Constant  Value=360
  Alpha 90<A<183 : Constant  Value=2
  Alpha 90<A<184 : Constant  Value=2
  Alpha 90<A<185 : Constant  Value=87
  Discrete-Time Integrator : DiscreteIntegrator  ExternalReset=rising  SampleTime=Ts  LimitOutput=on  UpperSaturationLimit=100000  LowerSaturationLimit=0  ICPrevOutput=DiscIntNeverNeededParam  ICPrevScaledInput=DiscIntNeverNeededParam
  Gain2 : Gain  Gain=1/Ts  SaturateOnIntegerOverflow=on  OutDataTypeStr=Inherit: Same as input  ParamDataTypeStr=Inherit: Same as input
  Logical Operator1 : Logic  Inputs=3
  Logical Operator2 : Logic  Operator=NOT  Inputs=3
  Product : Product  Inputs=*/  InputSameDT=on  SaturateOnIntegerOverflow=on  OutDataTypeStr=Inherit: Same as first input
  Product1 : Product  Inputs=**  InputSameDT=on  SaturateOnIntegerOverflow=on  OutDataTypeStr=Inherit: Same as first input
  Product2 : Product  Inputs=*/  InputSameDT=on  SaturateOnIntegerOverflow=on  OutDataTypeStr=Inherit: Same as first input
  Relational Operator1 : RelationalOperator  Operator=<=
  Relational Operator2 : RelationalOperator
  Relational Operator3 : RelationalOperator  Operator=<=
  Rounding Function1 : Rounding  Operator=round
  Rounding Function3 : Rounding  Operator=round
  Sample and Hold : spsSampleandHoldLib/Sample and Hold  ic=180  Ts=Ts
      settings: AttributesFormatString=IC = %<ic>
  Sum1 : Sum  Inputs=+-  InputSameDT=on  SaturateOnIntegerOverflow=on  OutDataTypeStr=Inherit: Same as first input
  Sum2 : Sum  Inputs=+--  InputSameDT=on  SaturateOnIntegerOverflow=on  OutDataTypeStr=Inherit: Same as first input
  Switch : Switch  Criteria=u2 > Threshold
  TCR +/- : Outport  VectorParamsAs1DForOutWhenUnconnected=off
  wires:
  Alpha 90<A<181/1 -> Sum1/2
  Ns/c/1 -> Product1/1, Product2/1
  Product1/1 -> Rounding Function1/1
  Alpha 90<A<182/1 -> Product/2
  Product/1 -> Product1/2
  Product2/1 -> Rounding Function3/1
  Alpha 90<A<183/1 -> Product2/2
  Sum1/1 -> Product/1, Relational Operator1/1
  Alpha 90<A<185/1 -> Relational Operator1/2
  Alpha/1 -> Sample and Hold/1
  Rounding Function1/1 -> Sum2/3, Switch/1
  Rounding Function3/1 -> Sum2/1, Switch/3
  Alpha 90<A<184/1 -> Sum2/2
  Relational Operator1/1 -> Switch/2
  Relational Operator3/1 -> Logical Operator1/3
  Discrete-Time Integrator/1 -> Relational Operator2/1, Relational Operator3/1
  Relational Operator2/1 -> Logical Operator1/2
  Logical Operator1/1 -> TCR +/-/1
  Gain2/1 -> Discrete-Time Integrator/1
  Switch/1 -> Relational Operator2/2
  Sum2/1 -> Relational Operator3/2
  Logical Operator2/1 -> Discrete-Time Integrator/2
  SqWave/1 -> Gain2/1, Logical Operator2/1, Logical Operator1/1
  Sync +/-/1 -> Sample and Hold/2
  Sample and Hold/1 -> Sum1/1

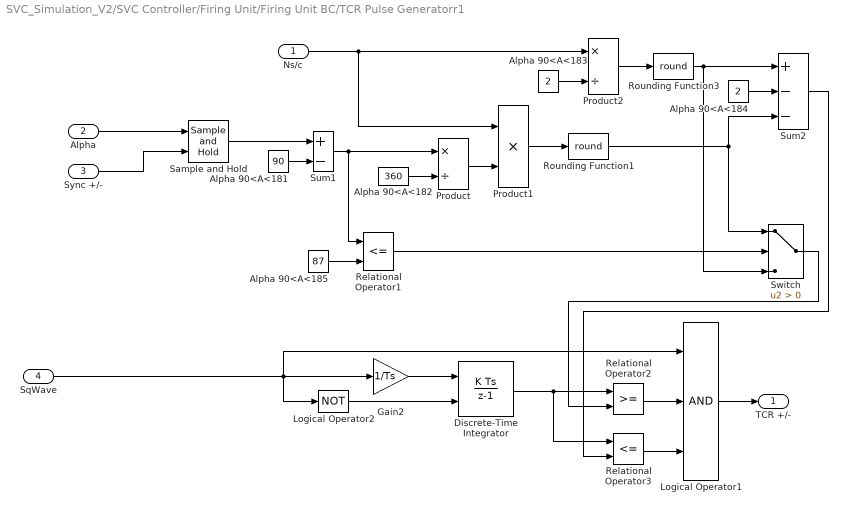
== system SVC_Simulation_V2/SVC Controller/Firing Unit/Firing Unit BC/TCR Pulse Generatorr1 ==
  Ns/c : Inport
  Alpha : Inport  Port=2  PortDimensions=1
  Sync +/- : Inport  Port=3  PortDimensions=1
  SqWave : Inport  Port=4  PortDimensions=1
  Alpha 90<A<181 : Constant  Value=90
  Alpha 90<A<182 : Constant  Value=360
  Alpha 90<A<183 : Constant  Value=2
  Alpha 90<A<184 : Constant  Value=2
  Alpha 90<A<185 : Constant  Value=87
  Discrete-Time Integrator : DiscreteIntegrator  ExternalReset=rising  SampleTime=Ts  LimitOutput=on  UpperSaturationLimit=100000  LowerSaturationLimit=0  ICPrevOutput=DiscIntNeverNeededParam  ICPrevScaledInput=DiscIntNeverNeededParam
  Gain2 : Gain  Gain=1/Ts  SaturateOnIntegerOverflow=on  OutDataTypeStr=Inherit: Same as input  ParamDataTypeStr=Inherit: Same as input
  Logical Operator1 : Logic  Inputs=3
  Logical Operator2 : Logic  Operator=NOT  Inputs=3
  Product : Product  Inputs=*/  InputSameDT=on  SaturateOnIntegerOverflow=on  OutDataTypeStr=Inherit: Same as first input
  Product1 : Product  Inputs=**  InputSameDT=on  SaturateOnIntegerOverflow=on  OutDataTypeStr=Inherit: Same as first input
  Product2 : Product  Inputs=*/  InputSameDT=on  SaturateOnIntegerOverflow=on  OutDataTypeStr=Inherit: Same as first input
  Relational Operator1 : RelationalOperator  Operator=<=
  Relational Operator2 : RelationalOperator
  Relational Operator3 : RelationalOperator  Operator=<=
  Rounding Function1 : Rounding  Operator=round
  Rounding Function3 : Rounding  Operator=round
  Sample and Hold : spsSampleandHoldLib/Sample and Hold  ic=180  Ts=Ts
      settings: AttributesFormatString=IC = %<ic>
  Sum1 : Sum  Inputs=+-  InputSameDT=on  SaturateOnIntegerOverflow=on  OutDataTypeStr=Inherit: Same as first input
  Sum2 : Sum  Inputs=+--  InputSameDT=on  SaturateOnIntegerOverflow=on  OutDataTypeStr=Inherit: Same as first input
  Switch : Switch  Criteria=u2 > Threshold
  TCR +/- : Outport  VectorParamsAs1DForOutWhenUnconnected=off
  wires:
  Alpha 90<A<181/1 -> Sum1/2
  Ns/c/1 -> Product1/1, Product2/1
  Product1/1 -> Rounding Function1/1
  Alpha 90<A<182/1 -> Product/2
  Product/1 -> Product1/2
  Product2/1 -> Rounding Function3/1
  Alpha 90<A<183/1 -> Product2/2
  Sum1/1 -> Product/1, Relational Operator1/1
  Alpha 90<A<185/1 -> Relational Operator1/2
  Alpha/1 -> Sample and Hold/1
  Rounding Function1/1 -> Sum2/3, Switch/1
  Rounding Function3/1 -> Sum2/1, Switch/3
  Alpha 90<A<184/1 -> Sum2/2
  Relational Operator1/1 -> Switch/2
  Relational Operator3/1 -> Logical Operator1/3
  Discrete-Time Integrator/1 -> Relational Operator2/1, Relational Operator3/1
  Relational Operator2/1 -> Logical Operator1/2
  Logical Operator1/1 -> TCR +/-/1
  Gain2/1 -> Discrete-Time Integrator/1
  Switch/1 -> Relational Operator2/2
  Sum2/1 -> Relational Operator3/2
  Logical Operator2/1 -> Discrete-Time Integrator/2
  SqWave/1 -> Gain2/1, Logical Operator2/1, Logical Operator1/1
  Sync +/-/1 -> Sample and Hold/2
  Sample and Hold/1 -> Sum1/1

== system SVC_Simulation_V2/SVC Controller/Firing Unit/Firing Unit BC/TCS Pulse Generator ==
  note: Note: Sync+ , Sync - and SqWave signals are inverted for TSC firing (i.e. positive thyristor is fired on negative peak voltage)
  SqWave : Inport  PortDimensions=1
  Sync + : Inport  Port=2  PortDimensions=1
  Sync - : Inport  Port=3  PortDimensions=1
  TSC_On : Inport  Port=4  PortDimensions=1
  Alpha1 : Constant  Value=FiringMode-1
  Delay : Delay  DelayLength=fix(1/FreqInit/Ts)
  Logical Operator1 : Logic  Operator=NOT
  Logical Operator10 : Logic  Operator=OR
  Logical Operator11 : Logic  Inputs=3
  Logical Operator12 : Logic
  Logical Operator13 : Logic
  Logical Operator14 : Logic  Operator=OR
  Logical Operator15 : Logic  Inputs=3
  Sample and Hold : spsSampleandHoldLib/Sample and Hold  ic=0  Ts=Ts
      settings: AttributesFormatString=IC = %<ic>
  Sample and Hold1 : spsSampleandHoldLib/Sample and Hold  ic=0  Ts=Ts
      settings: AttributesFormatString=IC = %<ic>
  TSC + : Outport  VectorParamsAs1DForOutWhenUnconnected=off
  TSC - : Outport  Port=2  VectorParamsAs1DForOutWhenUnconnected=off
  wires:
  Delay/1 -> Logical Operator14/2, Logical Operator10/2
  Logical Operator15/1 -> TSC -/1
  Logical Operator11/1 -> TSC +/1
  Logical Operator14/1 -> Logical Operator15/2
  Logical Operator10/1 -> Logical Operator11/2
  Logical Operator1/1 -> Logical Operator10/1
  SqWave/1 -> Logical Operator14/1, Logical Operator1/1
  Logical Operator12/1 -> Delay/1
  Alpha1/1 -> Logical Operator12/2
  Logical Operator13/1 -> Logical Operator12/1
  TSC_On/1 -> Sample and Hold1/1, Sample and Hold/1, Logical Operator15/3, Logical Operator11/3
  Sync -/1 -> Sample and Hold/2
  Sync +/1 -> Sample and Hold1/2
  Sample and Hold/1 -> Logical Operator13/1, Logical Operator11/1
  Sample and Hold1/1 -> Logical Operator13/2, Logical Operator15/1

== system SVC_Simulation_V2/SVC Controller/Firing Unit/Firing Unit BC/TCS Pulse Generator1 ==
  note: Note: Sync+ , Sync - and SqWave signals are inverted for TSC firing (i.e. positive thyristor is fired on negative peak voltage)
  SqWave : Inport  PortDimensions=1
  Sync + : Inport  Port=2  PortDimensions=1
  Sync - : Inport  Port=3  PortDimensions=1
  TSC_On : Inport  Port=4  PortDimensions=1
  Alpha1 : Constant  Value=FiringMode-1
  Delay : Delay  DelayLength=fix(1/FreqInit/Ts)
  Logical Operator1 : Logic  Operator=NOT
  Logical Operator10 : Logic  Operator=OR
  Logical Operator11 : Logic  Inputs=3
  Logical Operator12 : Logic
  Logical Operator13 : Logic
  Logical Operator14 : Logic  Operator=OR
  Logical Operator15 : Logic  Inputs=3
  Sample and Hold : spsSampleandHoldLib/Sample and Hold  ic=0  Ts=Ts
      settings: AttributesFormatString=IC = %<ic>
  Sample and Hold1 : spsSampleandHoldLib/Sample and Hold  ic=0  Ts=Ts
      settings: AttributesFormatString=IC = %<ic>
  TSC + : Outport  VectorParamsAs1DForOutWhenUnconnected=off
  TSC - : Outport  Port=2  VectorParamsAs1DForOutWhenUnconnected=off
  wires:
  Delay/1 -> Logical Operator14/2, Logical Operator10/2
  Logical Operator15/1 -> TSC -/1
  Logical Operator11/1 -> TSC +/1
  Logical Operator14/1 -> Logical Operator15/2
  Logical Operator10/1 -> Logical Operator11/2
  Logical Operator1/1 -> Logical Operator10/1
  SqWave/1 -> Logical Operator14/1, Logical Operator1/1
  Logical Operator12/1 -> Delay/1
  Alpha1/1 -> Logical Operator12/2
  Logical Operator13/1 -> Logical Operator12/1
  TSC_On/1 -> Sample and Hold1/1, Sample and Hold/1, Logical Operator15/3, Logical Operator11/3
  Sync -/1 -> Sample and Hold/2
  Sync +/1 -> Sample and Hold1/2
  Sample and Hold/1 -> Logical Operator13/1, Logical Operator11/1
  Sample and Hold1/1 -> Logical Operator13/2, Logical Operator15/1

== system SVC_Simulation_V2/SVC Controller/Firing Unit/Firing Unit BC/TCS Pulse Generator2 ==
  note: Note: Sync+ , Sync - and SqWave signals are inverted for TSC firing (i.e. positive thyristor is fired on negative peak voltage)
  SqWave : Inport  PortDimensions=1
  Sync + : Inport  Port=2  PortDimensions=1
  Sync - : Inport  Port=3  PortDimensions=1
  TSC_On : Inport  Port=4  PortDimensions=1
  Alpha1 : Constant  Value=FiringMode-1
  Delay : Delay  DelayLength=fix(1/FreqInit/Ts)
  Logical Operator1 : Logic  Operator=NOT
  Logical Operator10 : Logic  Operator=OR
  Logical Operator11 : Logic  Inputs=3
  Logical Operator12 : Logic
  Logical Operator13 : Logic
  Logical Operator14 : Logic  Operator=OR
  Logical Operator15 : Logic  Inputs=3
  Sample and Hold : spsSampleandHoldLib/Sample and Hold  ic=0  Ts=Ts
      settings: AttributesFormatString=IC = %<ic>
  Sample and Hold1 : spsSampleandHoldLib/Sample and Hold  ic=0  Ts=Ts
      settings: AttributesFormatString=IC = %<ic>
  TSC + : Outport  VectorParamsAs1DForOutWhenUnconnected=off
  TSC - : Outport  Port=2  VectorParamsAs1DForOutWhenUnconnected=off
  wires:
  Delay/1 -> Logical Operator14/2, Logical Operator10/2
  Logical Operator15/1 -> TSC -/1
  Logical Operator11/1 -> TSC +/1
  Logical Operator14/1 -> Logical Operator15/2
  Logical Operator10/1 -> Logical Operator11/2
  Logical Operator1/1 -> Logical Operator10/1
  SqWave/1 -> Logical Operator14/1, Logical Operator1/1
  Logical Operator12/1 -> Delay/1
  Alpha1/1 -> Logical Operator12/2
  Logical Operator13/1 -> Logical Operator12/1
  TSC_On/1 -> Sample and Hold1/1, Sample and Hold/1, Logical Operator15/3, Logical Operator11/3
  Sync -/1 -> Sample and Hold/2
  Sync +/1 -> Sample and Hold1/2
  Sample and Hold/1 -> Logical Operator13/1, Logical Operator11/1
  Sample and Hold1/1 -> Logical Operator13/2, Logical Operator15/1

== system SVC_Simulation_V2/SVC Controller/Firing Unit/Firing Unit CA/BL2 ==
  Freq : Inport  PortDimensions=1
  Constant1 : Constant  Value=0
  Constant2 : Constant  Value=1e-5
  Constant3 : Constant
  Gain : Gain  Gain=Ts  SaturateOnIntegerOverflow=on  OutDataTypeStr=Inherit: Same as input  ParamDataTypeStr=Inherit: Same as input
  Product : Product  Inputs=/*  InputSameDT=on  SaturateOnIntegerOverflow=on  OutDataTypeStr=Inherit: Same as first input
  Relational Operator1 : RelationalOperator  Operator=~=
  Switch : Switch  Threshold=0.5
  Ns/c : Outport  VectorParamsAs1DForOutWhenUnconnected=off
  wires:
  Product/1 -> Ns/c/1
  Freq/1 -> Gain/1
  Constant1/1 -> Relational Operator1/2
  Gain/1 -> Relational Operator1/1, Switch/1
  Constant2/1 -> Switch/3
  Relational Operator1/1 -> Switch/2
  Switch/1 -> Product/1
  Constant3/1 -> Product/2

== system SVC_Simulation_V2/SVC Controller/Firing Unit/Firing Unit CA/BL3 ==
  Freq : Inport  PortDimensions=1
  sin(wt) : Inport  Port=2  PortDimensions=1
  Bistable : spsBistableLib/Bistable  Qpriority=Set  ic=0  Ts=Ts
  Data Type Conversion : DataTypeConversion  SaturateOnIntegerOverflow=off  RndMeth=Floor
  Edge Detector : spsEdgeDetectorLib/Edge Detector  model=Rising  ic=0  Ts=Ts
  Edge Detector1 : spsEdgeDetectorLib/Edge Detector  model=Falling  ic=0  Ts=Ts
  Edge Detector2 : spsEdgeDetectorLib/Edge Detector  model=Rising  ic=0  Ts=Ts
  Edge Detector3 : spsEdgeDetectorLib/Edge Detector  model=Rising  ic=0  Ts=Ts
  Product2 : Product  InputSameDT=on  SaturateOnIntegerOverflow=on  OutDataTypeStr=Inherit: Same as first input
  Relational Operator : RelationalOperator  Operator=>
  Relational Operator2 : RelationalOperator  Operator=<
  Sum5 : Sum  Inputs=+-  InputSameDT=on  SaturateOnIntegerOverflow=on  OutDataTypeStr=Inherit: Same as first input
  Sum6 : Sum  InputSameDT=on  SaturateOnIntegerOverflow=on  OutDataTypeStr=Inherit: Same as first input
  Terminator : Terminator
  Trigonometric Function7 : Trigonometry
  alpha2 : Constant  Value=0
  alpha9 : Constant  Value=pi*Ts
  SqWave : Outport  VectorParamsAs1DForOutWhenUnconnected=off
  Sync + : Outport  Port=2  VectorParamsAs1DForOutWhenUnconnected=off
  Sync - : Outport  Port=3  VectorParamsAs1DForOutWhenUnconnected=off
  wires:
  Data Type Conversion/1 -> Edge Detector/1, Edge Detector1/1, SqWave/1
  Bistable/2 -> Terminator/1
  Edge Detector3/1 -> Bistable/2
  Edge Detector2/1 -> Bistable/1
  Edge Detector1/1 -> Sync -/1
  Edge Detector/1 -> Sync +/1
  Bistable/1 -> Data Type Conversion/1
  alpha9/1 -> Product2/1
  Product2/1 -> Trigonometric Function7/1
  Relational Operator2/1 -> Edge Detector3/1
  Relational Operator/1 -> Edge Detector2/1
  Sum6/1 -> Relational Operator2/2
  Sum5/1 -> Relational Operator/2
  alpha2/1 -> Sum6/1, Sum5/1
  Trigonometric Function7/1 -> Sum6/2, Sum5/2
  Freq/1 -> Product2/2
  sin(wt)/1 -> Relational Operator/1, Relational Operator2/1

== system SVC_Simulation_V2/SVC Controller/Firing Unit/Firing Unit CA/PLL sync on positive peak  ==
  note: Note: -sin( a ) * sin( b ) = 1/2 * cos( a+b ) - 1/2 * cos(a-b)
  note: Discrete 1-phase PLL
  note: Note: PLL synchronized on positive peak of input
  note: Pierre Giroux, Gilbert Sybille
      | Power System Laboratory, IREQ
      | Hydro-Quebec
  V(pu) : Inport
  Constant4 : Constant  Value=2*pi
  Discrete PI Controller : Subsystem  DialogController=POWERSYS.PowerSysDialog  mask(Discrete PI Controller){Kp=Kp, Ki=Ki, Par_Limits=[1.25  0.75]*2*pi*Finit, Init=2*pi*Finit, Ts=Ts}
      mask prompts: Kp "Proportional gain (Kp):"; Ki "Integral gain (Ki):"; Par_Limits "Output limits: [ Upper   Lower ]"; Init "Output initial value:"; Ts "Sample time:"
      mask help: This block implements a discrete PI controller.
      mask init:
      | UpperLimit=Par_Limits(1);
      | LowerLimit=Par_Limits(2);
      | power_initmask();
      mask Help: This block is part of a subset of blocks in the Extras library that does not have documentation associated with it, other than the block mask description.
      mask Display: disp('PI');
  Discrete-Time Integrator : DiscreteIntegrator  InitialCondition=(Phase_Init-90)*pi/180  SampleTime=Ts  ICPrevOutput=DiscIntNeverNeededParam  ICPrevScaledInput=DiscIntNeverNeededParam
  Gain10 : Gain  Gain=1/2/pi  SaturateOnIntegerOverflow=on  OutDataTypeStr=Inherit: Same as input  ParamDataTypeStr=Inherit: Same as input
  Gain12 : Gain  Gain=-1  SaturateOnIntegerOverflow=on  OutDataTypeStr=Inherit: Same as input  ParamDataTypeStr=Inherit: Same as input
  Math Function : Math  Operator=mod  SignedPower=on
  Mean (Variable Frequency)1 : spsMeanVariableFrequencyLib/Mean (Variable Frequency)  Finit=Finit  Fmin=45  Vinit=0  Ts=Ts
  Product1 : Product  InputSameDT=on  SaturateOnIntegerOverflow=on  OutDataTypeStr=Inherit: Same as first input
  Rate Limiter : RateLimiter  RisingSlewLimit=10  FallingSlewLimit=-10  SampleTimeMode=inherited  InitialCondition=Finit
  Second-Order Filter : spsSecondOrderFilterLib/Second-Order Filter  FilterType=Lowpass  Fo=25  Zeta=0.707  Ts=Ts  Initialize=on  Vac_Init="[0 0  Finit]"  Vdc_Init=Finit  PlotResponse=off  FreqRange=[1 500 1]
  Trigonometric Function6 : Trigonometry
  Unit Delay1 : UnitDelay  InitialCondition=Finit  SampleTime=Ts  HasFrameUpgradeWarning=on
      settings: AttributesFormatString=IC = %<InitialCondition>
  Freq : Outport  VectorParamsAs1DForOutWhenUnconnected=off
  wt : Outport  Port=2  VectorParamsAs1DForOutWhenUnconnected=off
  wires:
  Gain12/1 -> Product1/1
  V(pu)/1 -> Gain12/1
  Constant4/1 -> Math Function/2
  Discrete-Time Integrator/1 -> Math Function/1
  Product1/1 -> Mean (Variable Frequency)1/2
  Discrete PI Controller/1(Out) -> Discrete-Time Integrator/1, Gain10/1  "W"
  Gain10/1 -> Rate Limiter/1
  Rate Limiter/1 -> Second-Order Filter/1
  Second-Order Filter/1 -> Unit Delay1/1
  Trigonometric Function6/1 -> Product1/2
  Math Function/1 -> Trigonometric Function6/1, wt/1
  Unit Delay1/1 -> Mean (Variable Frequency)1/1, Freq/1
  Mean (Variable Frequency)1/1 -> Discrete PI Controller/1(Error)
